simulink model "reaction_pendulum"  (R2021b)
settings: Solver=FixedStepDiscrete  StartTime=0.0  StopTime=50  FixedStep=h  RelTol=1e-3  EnableMultiTasking=on
PreLoadFcn:
  | warning('off','MATLAB:dispatcher:InexactMatch');
InitFcn:
  | hwinit
values from neighbouring files (symbols this model uses):
  Ad = sys_d.A    [hwinit.m]
  Bd = sys_d.B    [hwinit.m]
  Cd = sys_d.C    [hwinit.m]
  connected = connect(est_mot, pendulum_sys, "u", ["theta", "phidot", "theta_dot"])    [interconnection.m]
  D = connected.D    [hwinit.m]    (also in linear_reaction_pendulum.m = zeros(2,1); motor_identification1.m = [0 0])
  h = 0.01    [hwinit.m]    (also in sines2_held.mat = 0.05; slow_squares.mat)
  J_theta = params.params(1)    [hwinit.m]    (also in nonlinear_estimation.m = 1)
  kt = params.params(5)    [hwinit.m]    (also in nonlinear_estimation.m = 0.591)
  mgL = params.params(6)    [hwinit.m]    (also in nonlinear_estimation.m = 1.029)
  R = 1 * diag(r)    [hwinit.m]
undefined symbols (not defined in the file or in its folder): Discrete, K, Time
libraries: simulink x2, ctrlSharedLib x1
settings Model: SimulationMode=external  ExtModeTrigDuration=100000  Creator=user  LastModifiedBy=qijunfeng
settings SolverCC: AlgebraicLoopSolver=TrustRegion
settings DataIOCC: SaveFormat=Array  SignalLoggingSaveFormat=ModelDataLogs  SaveOutput=off  SignalLogging=off  DSMLogging=off  SaveTime=off  ReturnWorkspaceOutputs=off
settings OptimizationCC: ExpressionDepthLimit=2147483647  LifeSpan=inf
settings DebuggingCC: UnderspecifiedInitializationDetection=Classic  MergeDetectMultiDrivingBlocksExec=none  SolverPrmCheckMsg=warning  FcnCallInpInsideContextMsg=warning  StateNameClashWarn=warning  SFUnexpectedBacktrackingDiag=warning  SFNoUnconditionalDefaultTransitionDiag=warning  SFExecutionAtInitializationDiag=none  SFMachineParentedDataDiag=warning  ArithmeticOperatorsInVariantConditions=warning
settings HardwareCC: ProdBitPerPointer=32  ProdBitPerSizeT=32  ProdBitPerPtrDiffT=32  ProdLargestAtomicFloat=None  ProdIntDivRoundTo=Undefined  ProdEndianess=Unspecified  ProdWordSize=32  ProdHWDeviceType=32-bit Generic
settings ModelReferenceCC: PropagateSignalLabelsOutOfModel=off
settings SFSimCC: SimUseLocalCustomCode=off  CustomCodeUndefinedFunction=UseInterfaceOnly
settings RTWCC: Description=rpend RTDAC/USB2 (Visual C/C++)  SystemTargetFile=rtcon_rpend_usb2.tlc  TemplateMakefile=rtcon_rpend_vc_usb2_x64.tmf  RTWUseLocalCustomCode=off
settings CodeAppCC: StateflowObjectComments=on
settings STFCustomTargetCC: ModelReferenceCompliant=off  CombineOutputUpdateFcns=on  MatFileLogging=on  GRTInterface=off  SystemTargetFile=rtcon_rpend_usb2.tlc
settings GRTTargetCC: TargetLangStandard=C89/C90 (ANSI)  ModelReferenceCompliant=off  ParMdlRefBuildCompliant=off  CompOptLevelCompliant=off  ConcurrentExecutionCompliant=off  CPPClassGenCompliant=off  UseToolchainInfoCompliant=off  ExtMode=on  ExtModeMexFile=rtcon_ext_comm
settings ConfigComp: CovMetricSettings=dw  CovSaveCumulativeToWorkspaceVar=on  CovSaveSingleToWorkspaceVar=on  CovExternalEMLEnable=off  CovSFcnEnable=off

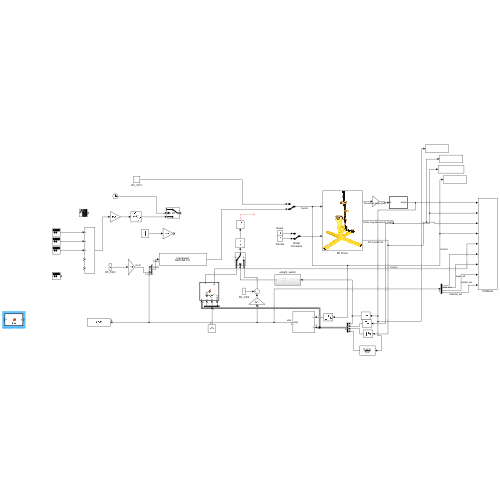
[thumbnail: Simulink's stored preview of the top-level diagram]
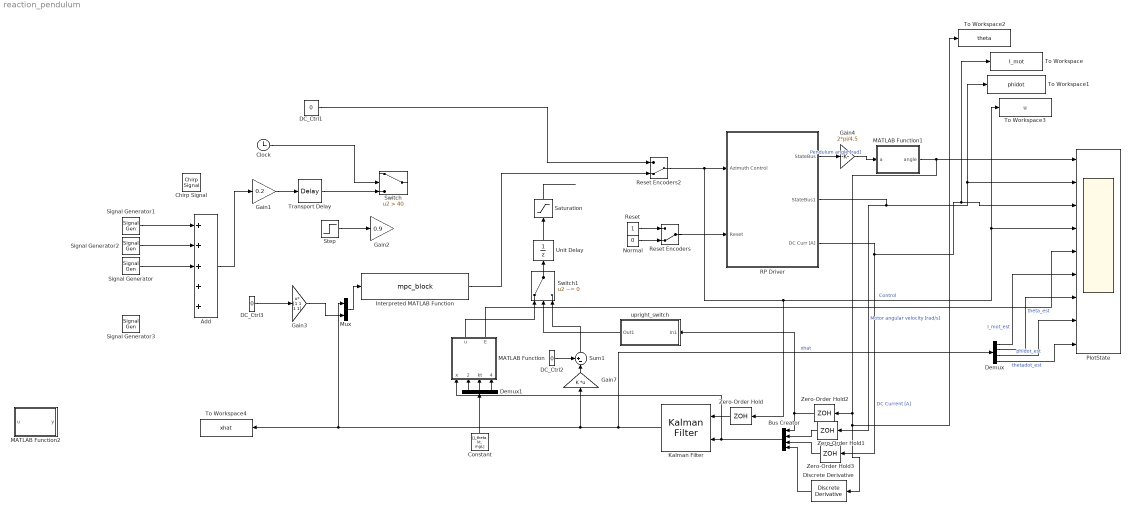
== system reaction_pendulum ==
  Add : Sum  Inputs=+++++
  Bus Creator : BusCreator  Inputs=4
  Chirp Signal : simulink/Sources/Chirp Signal  f1=0.05  T=20  f2=0.5
  Clock : Clock
  Constant : Constant  Value=[J_theta, kt, mgL]
  DC_Ctrl1 : Constant  Value=0
  DC_Ctrl2 : Constant  Value=0
  DC_Ctrl3 : Constant  Value=0
  Demux : Demux
  Demux1 : Demux  Outputs=3
  Discrete Derivative : simulink/Discrete/Discrete Derivative  gainval=1.0  ICPrevScaledInput=0.0  OutMin=-10  OutMax=10  OutDataType=fixdt(1, 16)  OutScaling=2^-10  DoSatur=off
  Gain1 : Gain  Gain=0.2
  Gain2 : Gain  Gain=0.9
  Gain3 : Gain  Gain=[1 1 1 1]  Multiplication=Matrix(u*K)
  Gain4 : Gain  Gain=2*pi/4.5
  Gain7 : Gain  Gain=K  Multiplication=Matrix(K*u)
  Interpreted MATLAB Function : MATLABFcn  MATLABFcn=mpc_block  OutputDimensions=1  OutputSignalType=real
  Kalman Filter : ctrlSharedLib/Kalman Filter  TimeDomain=Discrete-Time  UseCurrentEstimator=off  ModelSource=LTI State-Space Variable  ModelSourceVariable=c2d(connected,h)  A=Ad  B=Bd  C=Cd  D=D  NumberOfStates=4  NumberOfInputs=1  NumberOfOutputs=3  InitialEstimateSource=Dialog  X0=[0, 0, 0, 0]  P0=10  UseK=off  UseGH=off  NumberOfProcessNoiseInputs=1  G=1  TimeInvariantG=on  H=0  TimeInvariantH=on  Q=Q  TimeInvariantQ=on  R=R  TimeInvariantR=on  N=0  TimeInvariantN=on  AddInputPort=on  AddEnablePort=off  OutputEstimatedY=off  OutputP=off  Ts=-1
  MATLAB Function : MATLAB Function  TreatAsAtomicUnit=on
  MATLAB Function1 : MATLAB Function  TreatAsAtomicUnit=on
  MATLAB Function2 : MATLAB Function  TreatAsAtomicUnit=on
  Mux : Mux  Inputs=2
  Normal : Constant  Value=0
  PlotState : Scope  NumInputPorts=9
  RP Driver : Subsystem
      mask Display: image(imread('rwp.JPG'))
  Reset : Constant
  Reset Encoders : ManualSwitch  CurrentSetting=0
  Reset Encoders2 : ManualSwitch  CurrentSetting=0
  Saturation : Saturate  UpperLimit=1  LowerLimit=-1
  Signal Generator : SignalGenerator  WaveForm=square  Amplitude=0.3  Frequency=1/2
  Signal Generator1 : SignalGenerator  WaveForm=square  Amplitude=0.3  Frequency=1/5
  Signal Generator2 : SignalGenerator  WaveForm=square  Amplitude=0.5  Frequency=1/4
  Signal Generator3 : SignalGenerator  WaveForm=square  Amplitude=0.6  Frequency=3.29
  Step : Step  SampleTime=0
  Sum1 : Sum  Inputs=+-|
  Switch : Switch  Criteria=u2 > Threshold  Threshold=40
  Switch1 : Switch  Criteria=u2 ~= 0  Threshold=40
  To Workspace : ToWorkspace  VariableName=I_mot  SampleTime=-1
  To Workspace1 : ToWorkspace  VariableName=phidot  SampleTime=-1
  To Workspace2 : ToWorkspace  VariableName=theta  SampleTime=-1
  To Workspace3 : ToWorkspace  VariableName=u  SampleTime=-1
  To Workspace4 : ToWorkspace  VariableName=xhat  SampleTime=-1
  Transport Delay : TransportDelay
  Unit Delay : UnitDelay  SampleTime=-1  HasFrameUpgradeWarning=on
  Zero-Order Hold{,1..3} (4 alike) : ZeroOrderHold  SampleTime=h
  upright_switch : Subsystem
  wires:
  Normal/1 -> Reset Encoders/2
  Reset/1 -> Reset Encoders/1
  Reset Encoders/1 -> RP Driver/2(Reset)
  RP Driver/3(DC Curr [A]) -> Zero-Order Hold3/1, PlotState/3, To Workspace/1  "DC Current [A]"
  Reset Encoders2/1 -> RP Driver/1(Azimuth Control), To Workspace3/1, PlotState/4, Zero-Order Hold/1  "Control"
  RP Driver/2(StateBus1) -> To Workspace1/1, PlotState/2, Zero-Order Hold1/1  "Motor angular velocity [rad/s]"
  RP Driver/1(StateBus) -> Gain4/1  "Pendulum angle [rad]"
  Signal Generator/1 -> Add/3
  Signal Generator1/1 -> Add/1
  Signal Generator2/1 -> Add/2
  Clock/1 -> Switch/2
  Add/1 -> Gain1/1
  Step/1 -> Gain2/1
  Transport Delay/1 -> Switch/3
  Kalman Filter/1 -> Demux/1, Mux/1, To Workspace4/1, Gain7/1  "xhat"
  Gain1/1 -> Transport Delay/1
  Zero-Order Hold/1 -> Kalman Filter/1
  Bus Creator/1 -> MATLAB Function/1(x), Kalman Filter/2
  DC_Ctrl2/1 -> Sum1/1
  Demux/1 -> PlotState/6  "I_mot_est"
  Demux/2 -> PlotState/7  "theta_est"
  Demux/3 -> PlotState/8  "phidot_est"
  Demux/4 -> PlotState/9  "thetadot_est"
  Discrete Derivative/1 -> Bus Creator/4
  Gain4/1 -> MATLAB Function1/1(a)
  Gain7/1 -> Sum1/2
  DC_Ctrl1/1 -> Reset Encoders2/1
  Zero-Order Hold2/1 -> upright_switch/1(In1), Bus Creator/1
  Zero-Order Hold1/1 -> Bus Creator/2
  Zero-Order Hold3/1 -> Bus Creator/3
  Sum1/1 -> Switch1/3
  upright_switch/1(Out1) -> Switch1/2
  MATLAB Function/1(u) -> Switch1/1
  Saturation/1 -> ?
  Unit Delay/1 -> Saturation/1
  Switch1/1 -> Unit Delay/1
  MATLAB Function/2(E) -> PlotState/5
  MATLAB Function1/1(angle) -> Discrete Derivative/1, To Workspace2/1, Zero-Order Hold2/1, PlotState/1
  DC_Ctrl3/1 -> Gain3/1
  Interpreted MATLAB Function/1 -> Reset Encoders2/2
  Gain3/1 -> Mux/2
  Mux/1 -> Interpreted MATLAB Function/1
  Demux1/1 -> MATLAB Function/2(J_theta)
  Demux1/2 -> MATLAB Function/3(kt)
  Demux1/3 -> MATLAB Function/4(mgL)
  Constant/1 -> Demux1/1

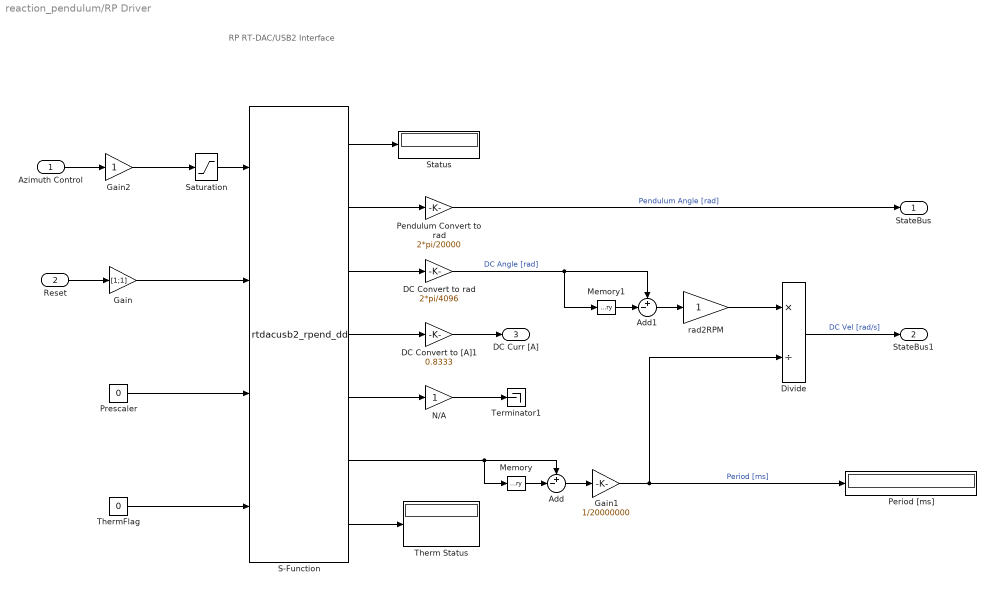
== system reaction_pendulum/RP Driver ==
  note: RP RT-DAC/USB2
      | Interface
  Azimuth Control : Inport
  Reset : Inport  Port=2
  Add : Sum  Inputs=+-|
  Add1 : Sum  Inputs=+-|
  DC Convert to [A]1 : Gain  Gain=0.8333  SaturateOnIntegerOverflow=on  OutDataTypeStr=Inherit: Same as input  ParamDataTypeStr=Inherit: Same as input
  DC Convert to rad : Gain  Gain=2*pi/4096  SaturateOnIntegerOverflow=on  OutDataTypeStr=Inherit: Same as input  ParamDataTypeStr=Inherit: Same as input
  Divide : Product  Inputs=*/
  Gain : Gain  Gain=[1;1]
  Gain1 : Gain  Gain=1/20000000
  Gain2 : Gain
  Memory : Memory
  Memory1 : Memory
  N/A : Gain  SaturateOnIntegerOverflow=on  OutDataTypeStr=Inherit: Same as input  ParamDataTypeStr=Inherit: Same as input
  Pendulum Convert to rad : Gain  Gain=2*pi/20000  SaturateOnIntegerOverflow=on  OutDataTypeStr=Inherit: Same as input  ParamDataTypeStr=Inherit: Same as input
  Period [ms] : Display
  Prescaler : Constant  Value=0
  S-Function : S-Function  FunctionName=rtdacusb2_rpend_dd  Parameters=1, h  SFunctionDeploymentMode=off  EnableBusSupport=off
  Saturation : Saturate  UpperLimit=1  LowerLimit=-1
  Status : Display
  Terminator1 : Terminator
  Therm Status : Display
  ThermFlag : Constant  Value=0
  rad2RPM : Gain  SaturateOnIntegerOverflow=on  OutDataTypeStr=Inherit: Same as input  ParamDataTypeStr=Inherit: Same as input
  StateBus : Outport  VectorParamsAs1DForOutWhenUnconnected=off
  StateBus1 : Outport  Port=2  VectorParamsAs1DForOutWhenUnconnected=off
  DC Curr [A] : Outport  Port=3  VectorParamsAs1DForOutWhenUnconnected=off
  wires:
  S-Function/7 -> Therm Status/1
  S-Function/5 -> N/A/1
  S-Function/4 -> DC Convert to [A]1/1
  ThermFlag/1 -> S-Function/4
  Prescaler/1 -> S-Function/3
  Gain/1 -> S-Function/2
  DC Convert to [A]1/1 -> DC Curr [A]/1
  Divide/1 -> StateBus1/1  "DC Vel [rad/s]"
  rad2RPM/1 -> Divide/1
  Add1/1 -> rad2RPM/1
  Memory1/1 -> Add1/2
  N/A/1 -> Terminator1/1
  S-Function/6 -> Add/1, Memory/1
  Gain2/1 -> Saturation/1
  Gain1/1 -> Period [ms]/1, Divide/2  "Period [ms]"
  Add/1 -> Gain1/1
  Memory/1 -> Add/2
  DC Convert to rad/1 -> Add1/1, Memory1/1  "DC Angle [rad]"
  S-Function/3 -> DC Convert to rad/1
  Pendulum Convert to rad/1 -> StateBus/1  "Pendulum Angle [rad]"
  S-Function/2 -> Pendulum Convert to rad/1
  S-Function/1 -> Status/1
  Saturation/1 -> S-Function/1
  Reset/1 -> Gain/1
  Azimuth Control/1 -> Gain2/1

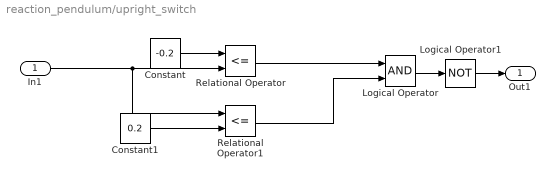
== system reaction_pendulum/upright_switch ==
  In1 : Inport
  Constant : Constant  Value=-0.2
  Constant1 : Constant  Value=0.2
  Logical Operator : Logic  AllPortsSameDT=off  OutDataTypeStr=boolean
  Logical Operator1 : Logic  Operator=NOT  AllPortsSameDT=off  OutDataTypeStr=boolean
  Relational Operator : RelationalOperator  Operator=<=  OutDataTypeStr=boolean  RndMeth=Simplest
  Relational Operator1 : RelationalOperator  Operator=<=  OutDataTypeStr=boolean  RndMeth=Simplest
  Out1 : Outport
  wires:
  In1/1 -> Relational Operator1/1, Relational Operator/2
  Constant/1 -> Relational Operator/1
  Constant1/1 -> Relational Operator1/2
  Relational Operator/1 -> Logical Operator/1
  Relational Operator1/1 -> Logical Operator/2
  Logical Operator/1 -> Logical Operator1/1
  Logical Operator1/1 -> Out1/1

== matlab function reaction_pendulum/MATLAB Function1 ==
  data: a input; angle output
function angle = fcn(a)
    b = a + pi;
    angle = mod(b, 2*pi);
    angle = angle - pi;

== matlab function reaction_pendulum/MATLAB Function ==
  data: x input; u output size=1; E output; J_theta input; kt input; mgL input
function [u, E] = swingup(x, J_theta, kt, mgL)
    E0 = 0.75;
    theta = x(1);
    thetadot = x(4);
    
    e_kin = 0.5 * J_theta * thetadot * thetadot;
    e_pot = 1.5 * mgL * (cos(theta) - 1);
    E = e_kin + e_pot;
%     E = -1;
%     E = min(E, 0);

    sign_term = sign(thetadot * cos(theta));
    k = 1;
    u = 1/kt * (E - E0) * sign_term;
end

== matlab function reaction_pendulum/MATLAB Function2 ==
  data: u input; y output
function y = fcn(u)

y = u;
